simulink model "s_trial_estudio_final"  (R2022b)
settings: Solver=VariableStepAuto  StartTime=0.0  StopTime=400  RelTol=1e-3
libraries: fuzblock x4, simulink x1
settings Model: Creator=sophy  LastModifiedBy=sophy

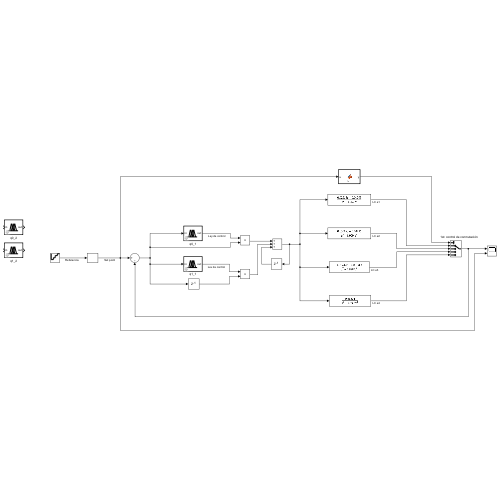
[thumbnail: Simulink's stored preview of the top-level diagram]
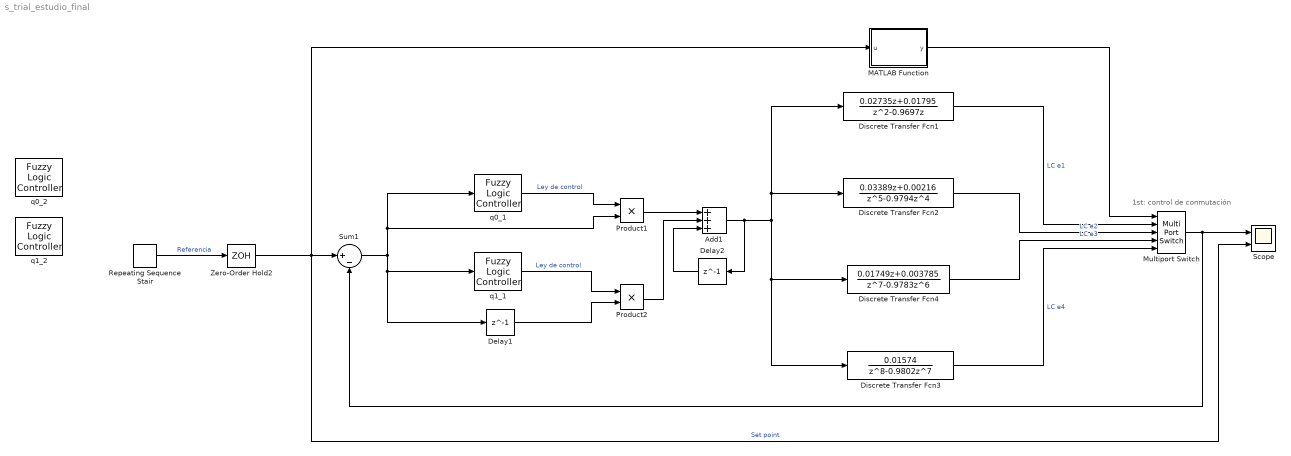
== system s_trial_estudio_final ==
  note: 1st: control de conmutación
  Add1 : Sum  Inputs=+++
  Delay1 : Delay  DelayLength=1
  Delay2 : Delay  DelayLength=1
  Discrete Transfer Fcn1 : DiscreteTransferFcn  Numerator=[0.02735 0.01795]  Denominator=[1 -0.9697 0]
  Discrete Transfer Fcn2 : DiscreteTransferFcn  Numerator=[0.03389 0.00216]  Denominator=[1 -0.9794 0 0 0 0]
  Discrete Transfer Fcn3 : DiscreteTransferFcn  Numerator=[0.01574]  Denominator=[1 -0.9802 0 0 0 0 0 0 0]
  Discrete Transfer Fcn4 : DiscreteTransferFcn  Numerator=[0.01749 0.003785]  Denominator=[1 -0.9783 0 0 0 0 0 0]
  MATLAB Function : MATLAB Function  TreatAsAtomicUnit=on
  Multiport Switch : MultiPortSwitch  Inputs=4  SaturateOnIntegerOverflow=off  InputSameDT=off
  Product1 : Product
  Product2 : Product
  Repeating Sequence Stair : simulink/Sources/Repeating Sequence Stair  OutValues=[20 30 40 50].'  tsamp=100  OutMin=[]  OutMax=[]  OutDataTypeStr=double  OutputDataTypeScalingMode=double  OutDataType=fixdt(0,8)  ConRadixGroup=Best Precision: Vector-wise  OutScaling=2^-12
  Scope : Scope  NumInputPorts=2
  Sum1 : Sum  Inputs=|+-
  Zero-Order Hold2 : ZeroOrderHold  SampleTime=0.2
  q0_1 : fuzblock/Fuzzy Logic  Controller  FIS=q0_e1  OutputSampleNumber=101  DataType=double  FuzzifiedInputs=off  RuleFiringStrengths=off  RuleOutputs=off  AggregatedOutputs=off  SimulateUsing=Interpreted execution  OutOfRangeInputValueMessage=warning  NoRuleFiredMessage=warning  EmptyOutputFuzzySetMessage=warning
  q0_2 : fuzblock/Fuzzy Logic  Controller  FIS=q0_e2  OutputSampleNumber=101  DataType=double  FuzzifiedInputs=off  RuleFiringStrengths=off  RuleOutputs=off  AggregatedOutputs=off  SimulateUsing=Interpreted execution  OutOfRangeInputValueMessage=warning  NoRuleFiredMessage=warning  EmptyOutputFuzzySetMessage=warning
  q1_1 : fuzblock/Fuzzy Logic  Controller  FIS=q1_e1  OutputSampleNumber=101  DataType=double  FuzzifiedInputs=off  RuleFiringStrengths=off  RuleOutputs=off  AggregatedOutputs=off  SimulateUsing=Interpreted execution  OutOfRangeInputValueMessage=warning  NoRuleFiredMessage=warning  EmptyOutputFuzzySetMessage=warning
  q1_2 : fuzblock/Fuzzy Logic  Controller  FIS=q1_e2  OutputSampleNumber=101  DataType=double  FuzzifiedInputs=off  RuleFiringStrengths=off  RuleOutputs=off  AggregatedOutputs=off  SimulateUsing=Interpreted execution  OutOfRangeInputValueMessage=warning  NoRuleFiredMessage=warning  EmptyOutputFuzzySetMessage=warning
  wires:
  Product2/1 -> Add1/2
  Sum1/1 -> q1_1/1, Delay1/1, q0_1/1, Product1/2
  Repeating Sequence Stair/1 -> Zero-Order Hold2/1  "Referencia"
  Add1/1 -> Delay2/1, Discrete Transfer Fcn1/1, Discrete Transfer Fcn2/1, Discrete Transfer Fcn3/1, Discrete Transfer Fcn4/1
  Discrete Transfer Fcn4/1 -> Multiport Switch/4  "LC e3"
  Discrete Transfer Fcn1/1 -> Multiport Switch/2  "LC e1"
  MATLAB Function/1(y) -> Multiport Switch/1
  Discrete Transfer Fcn3/1 -> Multiport Switch/5  "LC e4"
  Discrete Transfer Fcn2/1 -> Multiport Switch/3  "LC e2"
  Product1/1 -> Add1/1
  Delay2/1 -> Add1/3
  Delay1/1 -> Product2/2
  Multiport Switch/1 -> Sum1/2, Scope/1
  Zero-Order Hold2/1 -> Scope/2, MATLAB Function/1(u), Sum1/1  "Set point"
  q0_1/1 -> Product1/1  "Ley de control"
  q1_1/1 -> Product2/1  "Ley de control"

== matlab function s_trial_estudio_final/MATLAB Function ==
  data: u input; y output
function y = fcn(u)

if ((u>0)&&(u<=20)) % u = lo que entra = escalon
u = 1; % activar pin 1
end

if ((u>20)&&(u<=30))
u = 2; % activar pin 2
end 

if ((u>30)&&(u<=40))
u = 3; % activar pin 3
end 

if ((u>40)&&(u<=50))
u = 4; % activar pin 4
end 

y = u;
